simulink model "Practica7_Simulink"  (R2024a)
settings: Solver=VariableStepAuto  StartTime=0.0  StopTime=2.0  RelTol=1e-3
InitFcn:
  | R1=5e6;
  | R2=5e6;
  | R3=5e6;
  | C1=100e-9;
  | C2=100e-9;
settings Model: Creator=Manuel  LastModifiedBy=Manuel

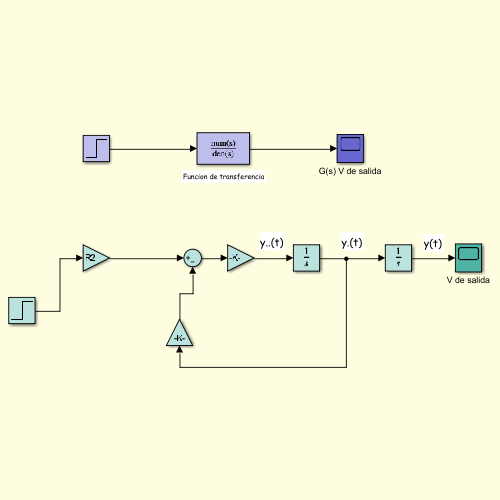
[thumbnail: Simulink's stored preview of the top-level diagram]
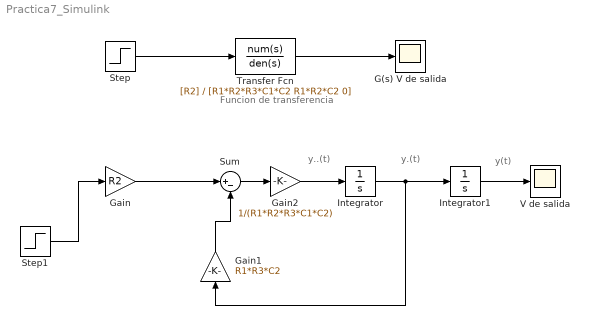
== system Practica7_Simulink ==
  note: y(t)
  note: y.(t)
  note: y..(t)
  note: Funcion de transferencia
  G(s) V de salida : Scope
  Gain : Gain  Gain=R2
  Gain1 : Gain  Gain=R1*R3*C2
  Gain2 : Gain  Gain=1/(R1*R2*R3*C1*C2)
  Integrator : Integrator
  Integrator1 : Integrator
  Step : Step  Time=0  SampleTime=0
  Step1 : Step  Time=0  SampleTime=0
  Sum : Sum  Inputs=|+-
  Transfer Fcn : TransferFcn  Numerator=[R2]  Denominator=[R1*R2*R3*C1*C2 R1*R2*C2 0]
  V de salida : Scope
  wires:
  Step/1 -> Transfer Fcn/1
  Transfer Fcn/1 -> G(s) V de salida/1
  Step1/1 -> Gain/1
  Gain/1 -> Sum/1
  Gain1/1 -> Sum/2
  Integrator/1 -> Gain1/1, Integrator1/1
  Gain2/1 -> Integrator/1
  Sum/1 -> Gain2/1
  Integrator1/1 -> V de salida/1
